simulink model "RELAY_TEST"  (Simulink 8.1)
settings: Solver=ode4  StartTime=0.0  StopTime=1.5  FixedStep=Ts  MaxStep=1e-3  RelTol=1e-3
model workspace (MAT data in the model file):
  op_snapshot1 : opcond.OperatingPoint (value not decoded)
PostLoadFcn:
  | Ts=100e-6; RELAY_TEST_init;
InitFcn:
  | Ts=100e-6; RELAY_TEST_init;
values from neighbouring files (symbols this model uses):
  cb_mech_delay = 5/60    (= 0.0833333333333)    [RELAY_TEST_init.m]
undefined symbols (not defined in the file or in its folder): cable_spec, Left, relay_par, type, V
libraries: rtlab x6, artemis x5, cables_lib x5, breaker_lib x3, relay_modbus_lib x3, rtio_generic_modbus x3, Load_lib x2, powerlib x2, ssn_lib x2, transformer_lib x2, powerlib_extras x1
settings Model: ARTEMISmethode_block_infos=$$__separator__$$RELAY_TEST/ARTEMIS Guide$$__separator__$$  Creator=RE25624  LastModifiedBy=re25624  BufferReuse=off
settings SolverCC: ZeroCrossAlgorithm=Adaptive
settings DataIOCC: ExternalInput=getinputstruct(op_snapshot1)  InitialState=getstatestruct(op_snapshot1)  LimitDataPoints=off  MaxDataPoints=90060  SignalLoggingSaveFormat=Dataset  SaveOutput=off  SignalLogging=off  DSMLogging=off  SaveTime=off  OutputSaveName=result
settings OptimizationCC: BlockReduction=off  OptimizeBlockIOStorage=off  BufferReuse=off  ExpressionFolding=off  LocalBlockOutputs=off
settings DebuggingCC: MaxConsecutiveZCsMsg=warning  IgnoredZcDiagnostic=none  SolverPrmCheckMsg=none  MultiTaskRateTransMsg=warning  FcnCallInpInsideContextMsg=EnableAllAsWarning  FrameProcessingCompatibilityMsg=error  ModelReferenceExtraNoncontSigs=warning  StrictBusMsg=None
settings ModelReferenceCC: UpdateModelReferenceTargets=IfOutOfDate
settings SFSimCC: SFSimEcho=off
settings GRTTargetCC: CodeReplacementLibrary=C89/C90 (ANSI)

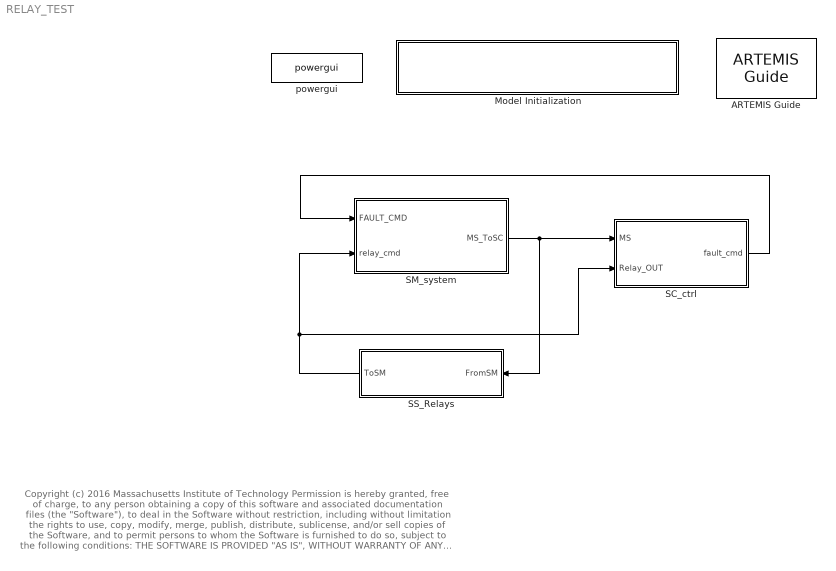
== system RELAY_TEST ==
  note: Copyright (c) 2016 Massachusetts Institute of Technology
      | Permission is hereby granted, free of charge, to any person obtaining a copy of this software and associated documentation files (the "Software"), to deal
      | in the Software without restriction, including without limitation the rights to use, copy, modify, merge, publish, distribute, sublicense, and/or sell copies of the
      | Software, and to permit persons to whom the Software is furnished to do so, subject to the following conditions:
      |
      | THE SOFTWARE IS PROVIDED "AS IS", WITHOUT WARRANTY OF ANY KIND, EXPRESS OR IMPLIED, INCLUDING BUT NOT LIMITED TO THE
      | WARRANTIES OF MERCHANTABILITY, FITNESS FOR A PARTICULAR PURPOSE AND NONINFRINGEMENT. IN NO EVENT SHALL THE AUTHORS
      | OR COPYRIGHT HOLDERS BE LIABLE FOR ANY CLAIM, DAMAGES OR OTHER LIABILITY, WHETHER IN AN ACTION OF CONTRACT, TORT OR
      | OTHERWISE, ARISING FROM, OUT OF OR IN CONNECTION WITH THE SOFTWARE OR THE USE OR OTHER DEALINGS IN THE SOFTWARE.
  ARTEMIS Guide : artemis/ARTEMIS/ARTEMIS Guide  Tag=FTSSmethode_opal_4hx0r99  Description=5.0_z1  lock=on  Ts=Ts  opt=art5  dyna=off  nb_perm=4  RT_fullcomp=off  ssn=on  ssn_itvc=off  ssn_ivic=off  ssn_ext=off  ssn_solver=Art5 with Backward Euler nodal interface  ssn_impulse=off  ssn_quasimpulse=off  ssn_impulse_loop=2  paraExtinctionThy=off  Thy_Impulse=on  dtc=Off  dtc_opt=normal  ao=on  simtype=off  ct_mac=off  lin_mov=off  lsp=[0.001 2]  spike_skip=Disabled  dtc_extra=1  dtc_sws=normal  dtc_pied=0.5  SPSRulesBlock=SPSRules  tre=on  ctmm=off  LF=off  dpl_type=ARTEMiS DPL  rlc_type=off  custom_type=off  para=on  ssn_ImpulseLoopBlockedStateUpdate=2  ssn_mov_iter_number=5  ssn_switch_iter_number=5
  Model Initialization : Subsystem  AncestorBlock=artemis/Tools /Misc/Model Initialization  mask(Model Functions){InitFcnX=Ts=100e-6; RELAY_TEST_init;, prel=off, posl=on, inif=on, strf=off}
      mask prompts: InitFcnX "Initialisation"; prel "Preload Function"; posl "PostLoad Function"; inif "InitFcn"; strf "StartFcn"
      mask init:
      | currentBlock = gcb;
      | root = bdroot(currentBlock);
      | 
      | 
      | if ~strcmp(get_param(root,'BlockDiagramType'),'library')
      |     if prel==1
      |         set_param(root, 'PreLoadFcn', InitFcnX);
      |     else
      |         set_param(root, 'PreLoadFcn', '');
      |     end
      |     if inif==1
      |         set_param(root, 'InitFcn', InitFcnX);
      |     else
      |         set_param(root, 'InitFcn', '');
      |     end
      |     if strf==1
      |         set_param(root, 'StartFcn', InitFcnX);
      |     else
      |         set_param(root, 'StartFcn', '');
      |     end
      |     if posl==1
      |         set_param(root, 'PostLoadFcn', InitFcnX);
      |     else
      |         set_param(root, 'PostLoadFcn', '');
      |     end
      | end
      | 
      | pos = get_param(currentBlock, 'Position');
      | width = pos(3) - pos(1); height = pos(4) - pos(2);
      | txt = [ upper(root) '\n' '- InitFcn. . . . . '  get_param(root, 'InitFcn') ];
      settings: CopyFcn=set_param(gcb,'LinkStatus','inactive')
      mask Display: text(5, height*0.5, txt, 'horizontalAlignment', 'left', 'verticalAlignment', 'middle') ;
  SC_ctrl : Subsystem
  SM_system : Subsystem
  SS_Relays : Subsystem
  powergui : powerlib/powergui  Priority=2  SimulationMode=Discrete  SolverType=Tustin  SampleTime=Ts  frequency=60  SPID=off  DisableSnubberDevices=off  DisableRonSwitches=off  DisableVfSwitches=off  SwTol=0  Interpol=off  DisplayEquations=off  frequencyindice=0  Pbase=100e6  ErrMax=1e-4  Iterations=50  UnitsV=kV  UnitsW=MW  FunctionMessages=off  echomessages=off  HookPort=off  EnableUseOfTLC=off  x0status=blocks  RestoreLinks=warning  ResistiveCurrentMeasurement=off  Frange=logspace(0,3,50)  Ylog=off  Xlog=off  ShowGrid=off  save=off  variable=ZData  structure=0  ZoomFFT=on  StartTime=0.0  cycles=2  DisplayStyle=off  fundamental=60  FreqAxis=off  MaxFrequency=1000  frequencyindicesteady=1  RmsSteady=1  display=off  Ts=0  methode=off
  wires:
  SM_system/1(MS_ToSC) -> SS_Relays/1(FromSM), SC_ctrl/1(MS)
  SS_Relays/1(ToSM) -> SM_system/2(relay_cmd), SC_ctrl/2(Relay_OUT)
  SC_ctrl/1(fault_cmd) -> SM_system/1(FAULT_CMD)

== system RELAY_TEST/Model Initialization ==

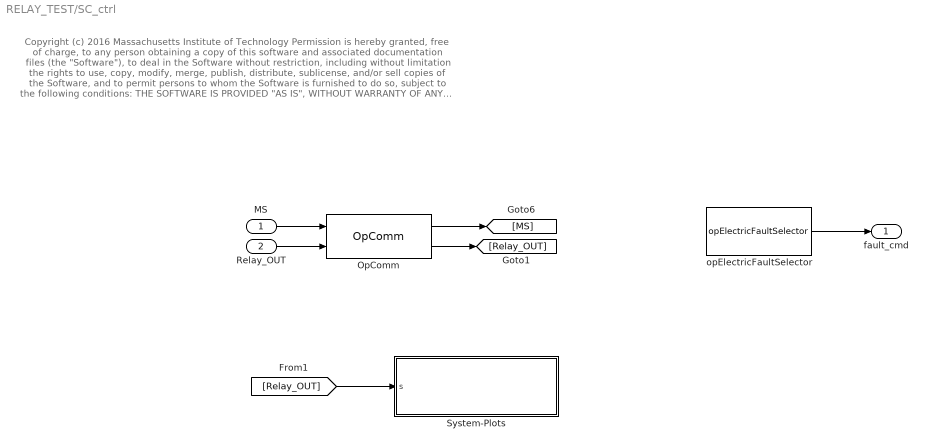
== system RELAY_TEST/SC_ctrl ==
  note: Copyright (c) 2016 Massachusetts Institute of Technology
      | Permission is hereby granted, free of charge, to any person obtaining a copy of this software and associated documentation files (the "Software"), to deal
      | in the Software without restriction, including without limitation the rights to use, copy, modify, merge, publish, distribute, sublicense, and/or sell copies of the
      | Software, and to permit persons to whom the Software is furnished to do so, subject to the following conditions:
      |
      | THE SOFTWARE IS PROVIDED "AS IS", WITHOUT WARRANTY OF ANY KIND, EXPRESS OR IMPLIED, INCLUDING BUT NOT LIMITED TO THE
      | WARRANTIES OF MERCHANTABILITY, FITNESS FOR A PARTICULAR PURPOSE AND NONINFRINGEMENT. IN NO EVENT SHALL THE AUTHORS
      | OR COPYRIGHT HOLDERS BE LIABLE FOR ANY CLAIM, DAMAGES OR OTHER LIABILITY, WHETHER IN AN ACTION OF CONTRACT, TORT OR
      | OTHERWISE, ARISING FROM, OUT OF OR IN CONNECTION WITH THE SOFTWARE OR THE USE OR OTHER DEALINGS IN THE SOFTWARE.
  MS : Inport
  Relay_OUT : Inport  Port=2
  OpComm : rtlab/OpComm  nbport=2  groupe_acq=1  subsys_rate=0  st=0  Synchronization=on  Interpolation=on  Threshold=1.0  Missed_Data=off  Sim_Time=off  Samples=off  dynSigOut=off  from_console=0  warning_done=off  writeOpCommFile=off  Offset=off
  System-Plots : Subsystem
  opElectricFaultSelector : artemis/Tools /POW faults/opElectricFaultSelector  phase_a=on  phase_b=on  phase_c=on  gnd_fault=on  Tacq=1  Tst=[0.1 0 10]  enable_POW=on  angle_POW=[15 0 10]  Tdr="[10.5 0  20]"  fault_location_menu=location 2  T_init=0
  fault_cmd : Outport
  wires:
  OpComm/1 -> [MS]
  MS/1 -> OpComm/1
  OpComm/2 -> [Relay_OUT]
  Relay_OUT/1 -> OpComm/2
  opElectricFaultSelector/1 -> fault_cmd/1
  [Relay_OUT] -> System-Plots/1(s)

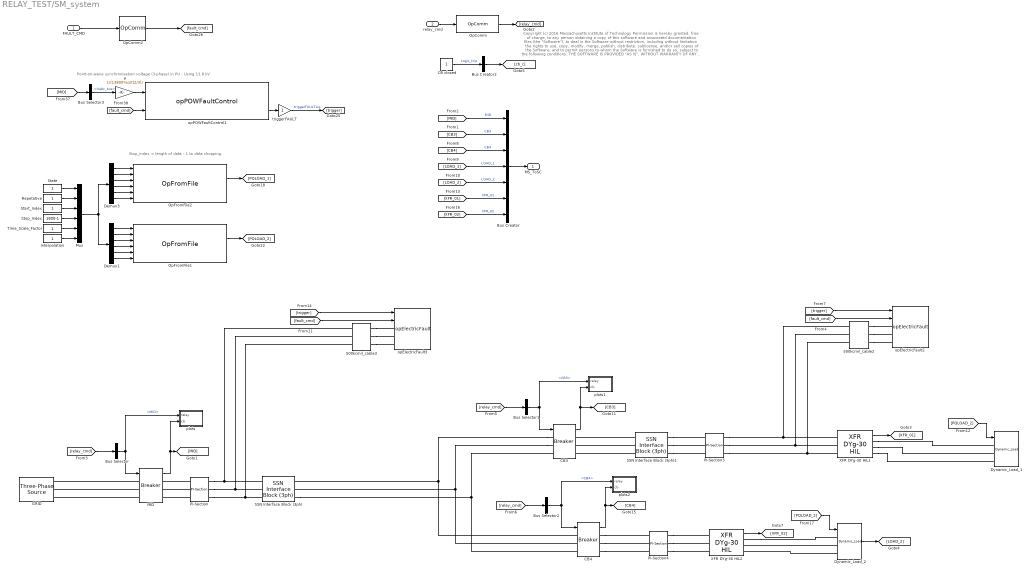
== system RELAY_TEST/SM_system ==
  note: Copyright (c) 2016 Massachusetts Institute of Technology
      | Permission is hereby granted, free of charge, to any person obtaining a copy of this software and associated documentation files (the "Software"), to deal
      | in the Software without restriction, including without limitation the rights to use, copy, modify, merge, publish, distribute, sublicense, and/or sell copies of the
      | Software, and to permit persons to whom the Software is furnished to do so, subject to the following conditions:
      |
      | THE SOFTWARE IS PROVIDED "AS IS", WITHOUT WARRANTY OF ANY KIND, EXPRESS OR IMPLIED, INCLUDING BUT NOT LIMITED TO THE
      | WARRANTIES OF MERCHANTABILITY, FITNESS FOR A PARTICULAR PURPOSE AND NONINFRINGEMENT. IN NO EVENT SHALL THE AUTHORS
      | OR COPYRIGHT HOLDERS BE LIABLE FOR ANY CLAIM, DAMAGES OR OTHER LIABILITY, WHETHER IN AN ACTION OF CONTRACT, TORT OR
      | OTHERWISE, ARISING FROM, OUT OF OR IN CONNECTION WITH THE SOFTWARE OR THE USE OR OTHER DEALINGS IN THE SOFTWARE
  note: Stop_index = length of data - 1 to data chopping
  note: Point-on-wave synchronisation voltage (3-phase) in PU - Using 13.8 kV
  FAULT_CMD : Inport
  relay_cmd : Inport  Port=2
  500kcmil_cable2 : cables_lib/500kcmil_cable  length=1  par_sets=1
  500kcmil_cable3 : cables_lib/500kcmil_cable  length=1  par_sets=1
  Bus Creator : BusCreator  Inputs=7
  Bus Creator2 : BusCreator  Inputs=1
  Bus Selector : BusSelector  OutputSignals=MID
  Bus Selector1 : BusSelector  OutputSignals=CB3
  Bus Selector2 : BusSelector  OutputSignals=CB4
  Bus Selector3 : BusSelector  OutputSignals=Vabc_bus
  CB closed : Constant
  CB3 : breaker_lib/Breaker  Ts=Ts  mech_delays=[cb_mech_delay(1,:)]
  CB4 : breaker_lib/Breaker  Ts=Ts  mech_delays=[cb_mech_delay(1,:)]
  Demux1 : Demux  Outputs=6
  Demux3 : Demux  Outputs=6
  Dynamic_Load_1 : Load_lib/Dynamic_Load  V=4160  Ts=Ts
  Dynamic_Load_2 : Load_lib/Dynamic_Load  V=480  Ts=Ts
  GRID : powerlib/Electrical Sources/Three-Phase Source  Voltage=13800  PhaseAngle=0  Frequency=60  InternalConnection=Yg  SpecifyImpedance=on  Resistance=0.8929  Inductance=16.58e-3  ShortCircuitLevel=375e6  BaseVoltage=13800  XRratio=4.6  BusType=swing  Pref=0  Qref=0  Qmin=-inf  Qmax=inf
  "Interpolation " : Constant
  MID : breaker_lib/Breaker  Ts=Ts  mech_delays=[cb_mech_delay(1,:)]
  Mux : Mux  Inputs=6
  OpComm : rtlab/OpComm  nbport=1  groupe_acq=1  subsys_rate=0  st=0  Synchronization=on  Interpolation=on  Threshold=1.0  Missed_Data=off  Sim_Time=off  Samples=off  dynSigOut=off  from_console=0  warning_done=off  writeOpCommFile=off  Offset=off
  OpComm2 : rtlab/OpComm  nbport=1  groupe_acq=1  subsys_rate=0  st=0  Synchronization=on  Interpolation=on  Threshold=1.0  Missed_Data=off  Sim_Time=off  Samples=off  dynSigOut=off  from_console=1  warning_done=off  writeOpCommFile=off  Offset=off
  OpFromFile1 : rtlab/DataLogging/OpFromFile  filename_mode=Static (same filename all the time)  reload_mode=Next time model is paused (Real-Time)  init_file_id=0  filename=one_min_data.mat  rtpath='./'  nrtpath='.\'  sample_time=0
  OpFromFile2 : rtlab/DataLogging/OpFromFile  filename_mode=Static (same filename all the time)  reload_mode=Next time model is paused (Real-Time)  init_file_id=0  filename=one_min_data.mat  rtpath='./'  nrtpath='.\'  sample_time=0
  PI-Section : cables_lib/PI-Section  cable_spec=[cable_spec(13, :)]  line_length=5500  parallel_sets=1
  PI-Section3 : cables_lib/PI-Section  cable_spec=[cable_spec(13, :)]  line_length=1500  parallel_sets=1
  PI-Section4 : cables_lib/PI-Section  cable_spec=[cable_spec(13, :)]  line_length=7000  parallel_sets=1
  "Repetative " : Constant
  SSN Interface Block (3ph) : ssn_lib/SSN Interface Block (3ph)  nb_phase=3  nb_port=2  p1_type=V-type(Left)  p2_type=V-type (Right)  p3_type=V-type(Left)  p4_type=V-type(Left)  p5_type=V-type(Left)  p6_type=V-type(Left)  p7_type=V-type(Left)  p8_type=V-type(Left)  p9_type=V-type(Left)  p10_type=V-type(Left)  p11_type=V-type(Left)  p12_type=V-type(Left)  p13_type=V-type(Left)  p14_type=V-type(Left)  p15_type=V-type(Left)  p16_type=V-type(Left)  I_port_shunt_resistance=1e9
  SSN Interface Block (3ph)1 : ssn_lib/SSN Interface Block (3ph)  nb_phase=3  nb_port=2  p1_type=V-type(Left)  p2_type=V-type (Right)  p3_type=V-type(Left)  p4_type=V-type(Left)  p5_type=V-type(Left)  p6_type=V-type(Left)  p7_type=V-type(Left)  p8_type=V-type(Left)  p9_type=V-type(Left)  p10_type=V-type(Left)  p11_type=V-type(Left)  p12_type=V-type(Left)  p13_type=V-type(Left)  p14_type=V-type(Left)  p15_type=V-type(Left)  p16_type=V-type(Left)  I_port_shunt_resistance=1e9
  "Start_Index " : Constant
  "State " : Constant
  "Stop_Index " : Constant  Value=1800-1
  "Time_Scale_Factor " : Constant
  XFR DYg-30 HIL1 : transformer_lib/XFR DYg-30 HIL  Rating=3750  Vp=13800  Vs=4160  Z=4.75  XR=11.4
  XFR DYg-30 HIL2 : transformer_lib/XFR DYg-30 HIL  Rating=2500  Vp=13800  Vs=480  Z=5.75  XR=6.6
  a : Gain  Gain=1/(13800*sqrt(2/3))
  opElectricFault2 : artemis/Tools /POW faults/opElectricFault  FaultLocation=location 2  FaultResistance=0.0001  GroundResistance=0.0001  InitialStates=[0 0 0]  SnubberResistance=1e6  SnubberCapacitance=inf
  opElectricFault3 : artemis/Tools /POW faults/opElectricFault  FaultLocation=location 1  FaultResistance=0.0001  GroundResistance=0.0001  InitialStates=[0 0 0]  SnubberResistance=1e6  SnubberCapacitance=inf
  opPOWFaultControl1 : artemis/Tools /POW faults/opPOWFaultControl  Ts=Ts  usePLL=off  Fgrid=60  PLL_k=[180 3200 1]  vol_sel=1: rising zero-corssing  SyncPhase_menu=A  T_acq=0.8
  plots : Subsystem
  plots1 : Subsystem
  plots2 : Subsystem
  triggerFAULT : Gain
  MS_ToSC : Outport
  wires:
  MID/1 -> plots/2(cb), [MID]
  Bus Creator/1 -> MS_ToSC/1
  OpComm/1 -> [relay_cmd]
  relay_cmd/1 -> OpComm/1
  XFR DYg-30 HIL1/1 -> [XFR_01]
  "Stop_Index "/1 -> Mux/4
  Demux1/2 -> OpFromFile1/2
  Demux1/5 -> OpFromFile1/5
  OpFromFile1/2 -> [PQLOAD_2]
  "Interpolation "/1 -> Mux/6
  Demux1/4 -> OpFromFile1/4
  Demux1/1 -> OpFromFile1/1
  Demux1/6 -> OpFromFile1/6
  Demux1/3 -> OpFromFile1/3
  "Start_Index "/1 -> Mux/3
  "Time_Scale_Factor "/1 -> Mux/5
  "Repetative "/1 -> Mux/2
  "State "/1 -> Mux/1
  XFR DYg-30 HIL2/1 -> [XFR_02]
  Bus Creator2/1 -> [cb_c]
  CB closed/1 -> Bus Creator2/1  "Logic_trip"
  [XFR_02] -> Bus Creator/7  "XFR_02"
  [LOAD_2] -> Bus Creator/5  "LOAD_2"
  [XFR_01] -> Bus Creator/6  "XFR_01"
  [MID] -> Bus Creator/1  "MID"
  [CB4] -> Bus Creator/3  "CB4"
  [CB3] -> Bus Creator/2  "CB3"
  [LOAD_1] -> Bus Creator/4  "LOAD_1"
  Demux3/2 -> OpFromFile2/2
  Demux3/5 -> OpFromFile2/5
  OpFromFile2/2 -> [PQLOAD_1]
  Demux3/4 -> OpFromFile2/4
  Demux3/1 -> OpFromFile2/1
  Demux3/6 -> OpFromFile2/6
  Demux3/3 -> OpFromFile2/3
  Mux/1 -> Demux1/1, Demux3/1
  [relay_cmd] -> Bus Selector/1
  Bus Selector/1 -> plots/1(relay), MID/1  "<MID>"
  [relay_cmd] -> Bus Selector1/1
  [relay_cmd] -> Bus Selector2/1
  [fault_cmd] -> opPOWFaultControl1/2
  opPOWFaultControl1/2 -> triggerFAULT/1
  triggerFAULT/1 -> [trigger]  "triggerFAULTsig"
  [MID] -> Bus Selector3/1
  Bus Selector3/1 -> a/1  "<Vabc_bus>"
  a/1 -> opPOWFaultControl1/1
  OpComm2/1 -> [fault_cmd]
  FAULT_CMD/1 -> OpComm2/1
  [fault_cmd] -> opElectricFault2/2
  [trigger] -> opElectricFault2/1
  [fault_cmd] -> opElectricFault3/2
  [trigger] -> opElectricFault3/1
  CB3/1 -> [CB3], plots1/2(cb)
  Bus Selector1/1 -> CB3/1, plots1/1(relay)  "<CB3>"
  CB4/1 -> plots2/2(cb), [CB4]
  Bus Selector2/1 -> CB4/1, plots2/1(relay)  "<CB4>"
  Dynamic_Load_2/1 -> [LOAD_2]
  [PQLOAD_2] -> Dynamic_Load_2/1
  [PQLOAD_2] -> Dynamic_Load_1/1
  connections:
  CB4/RConn2 -- PI-Section4/LConn2
  CB4/RConn1 -- PI-Section4/LConn1
  CB4/RConn3 -- PI-Section4/LConn3
  PI-Section4/RConn1 -- XFR DYg-30 HIL2/LConn1
  PI-Section4/RConn2 -- XFR DYg-30 HIL2/LConn2
  PI-Section4/RConn3 -- XFR DYg-30 HIL2/LConn3
  PI-Section3/RConn2 -- 500kcmil_cable2/LConn2 -- XFR DYg-30 HIL1/LConn2
  PI-Section3/RConn3 -- 500kcmil_cable2/LConn3 -- XFR DYg-30 HIL1/LConn3
  PI-Section3/RConn1 -- 500kcmil_cable2/LConn1 -- XFR DYg-30 HIL1/LConn1
  500kcmil_cable2/RConn2 -- opElectricFault2/LConn2
  500kcmil_cable2/RConn1 -- opElectricFault2/LConn1
  500kcmil_cable2/RConn3 -- opElectricFault2/LConn3
  500kcmil_cable3/RConn2 -- opElectricFault3/LConn2
  500kcmil_cable3/RConn1 -- opElectricFault3/LConn1
  500kcmil_cable3/RConn3 -- opElectricFault3/LConn3
  SSN Interface Block (3ph)1/RConn2 -- PI-Section3/LConn2
  SSN Interface Block (3ph)1/RConn1 -- PI-Section3/LConn1
  SSN Interface Block (3ph)1/RConn3 -- PI-Section3/LConn3
  SSN Interface Block (3ph)1/LConn3 -- CB3/RConn3
  SSN Interface Block (3ph)1/LConn1 -- CB3/RConn1
  SSN Interface Block (3ph)1/LConn2 -- CB3/RConn2
  500kcmil_cable3/LConn1 -- SSN Interface Block (3ph)/LConn1 -- PI-Section/RConn1
  500kcmil_cable3/LConn2 -- SSN Interface Block (3ph)/LConn2 -- PI-Section/RConn2
  500kcmil_cable3/LConn3 -- SSN Interface Block (3ph)/LConn3 -- PI-Section/RConn3
  SSN Interface Block (3ph)/RConn3 -- CB3/LConn3 -- CB4/LConn3
  CB3/LConn1 -- SSN Interface Block (3ph)/RConn1 -- CB4/LConn1
  CB3/LConn2 -- SSN Interface Block (3ph)/RConn2 -- CB4/LConn2
  Dynamic_Load_2/LConn2 -- XFR DYg-30 HIL2/RConn2
  Dynamic_Load_2/LConn3 -- XFR DYg-30 HIL2/RConn3
  Dynamic_Load_2/LConn1 -- XFR DYg-30 HIL2/RConn1
  XFR DYg-30 HIL1/RConn1 -- Dynamic_Load_1/LConn1
  XFR DYg-30 HIL1/RConn2 -- Dynamic_Load_1/LConn2
  XFR DYg-30 HIL1/RConn3 -- Dynamic_Load_1/LConn3
  PI-Section/LConn2 -- MID/RConn2
  PI-Section/LConn1 -- MID/RConn1
  PI-Section/LConn3 -- MID/RConn3
  MID/LConn1 -- GRID/RConn1
  MID/LConn2 -- GRID/RConn2
  MID/LConn3 -- GRID/RConn3

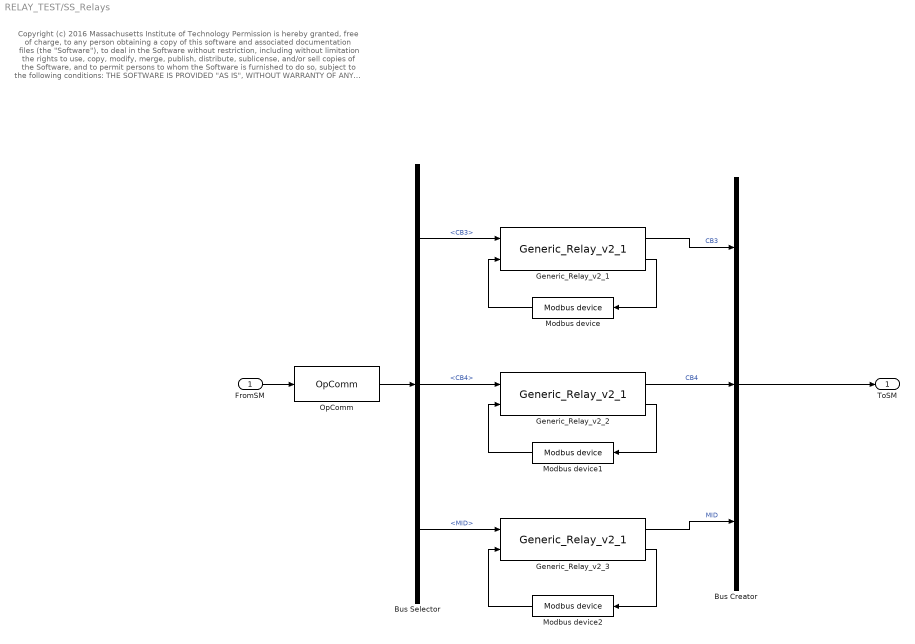
== system RELAY_TEST/SS_Relays ==
  note: Copyright (c) 2016 Massachusetts Institute of Technology
      | Permission is hereby granted, free of charge, to any person obtaining a copy of this software and associated documentation files (the "Software"), to deal
      | in the Software without restriction, including without limitation the rights to use, copy, modify, merge, publish, distribute, sublicense, and/or sell copies of the
      | Software, and to permit persons to whom the Software is furnished to do so, subject to the following conditions:
      |
      | THE SOFTWARE IS PROVIDED "AS IS", WITHOUT WARRANTY OF ANY KIND, EXPRESS OR IMPLIED, INCLUDING BUT NOT LIMITED TO THE
      | WARRANTIES OF MERCHANTABILITY, FITNESS FOR A PARTICULAR PURPOSE AND NONINFRINGEMENT. IN NO EVENT SHALL THE AUTHORS
      | OR COPYRIGHT HOLDERS BE LIABLE FOR ANY CLAIM, DAMAGES OR OTHER LIABILITY, WHETHER IN AN ACTION OF CONTRACT, TORT OR
      | OTHERWISE, ARISING FROM, OUT OF OR IN CONNECTION WITH THE SOFTWARE OR THE USE OR OTHER DEALINGS IN THE SOFTWARE
  FromSM : Inport
  Bus Creator : BusCreator  Inputs=3
  Bus Selector : BusSelector  OutputSignals=CB3,CB4,MID
  Generic_Relay_v2_1 : relay_modbus_lib/Generic_Relay_v2_1  Ts=Ts  relay_settings=[relay_par(1,:)]
  Generic_Relay_v2_2 : relay_modbus_lib/Generic_Relay_v2_1  Ts=Ts  relay_settings=[relay_par(2,:)]
  Generic_Relay_v2_3 : relay_modbus_lib/Generic_Relay_v2_1  Ts=Ts  relay_settings=[relay_par(1,:)]
  Modbus device : rtio_generic_modbus/Modbus device  conf_name=F1_relay_cfg1.opal  conf_name_mask=F1_relay_cfg1.xls  sample_time=Ts
  Modbus device1 : rtio_generic_modbus/Modbus device  conf_name=F1_relay_cfg2.opal  conf_name_mask=F1_relay_cfg2.xls  sample_time=Ts
  Modbus device2 : rtio_generic_modbus/Modbus device  conf_name=F1_relay_cfg3.opal  conf_name_mask=F1_relay_cfg3.xls  sample_time=Ts
  OpComm : rtlab/OpComm  nbport=1  groupe_acq=1  subsys_rate=0  st=0  Synchronization=on  Interpolation=on  Threshold=1.0  Missed_Data=off  Sim_Time=off  Samples=off  dynSigOut=off  from_console=0  warning_done=off  writeOpCommFile=off  Offset=off
  ToSM : Outport
  wires:
  OpComm/1 -> Bus Selector/1
  FromSM/1 -> OpComm/1
  Generic_Relay_v2_1/1 -> Bus Creator/1  "CB3"
  Generic_Relay_v2_2/1 -> Bus Creator/2  "CB4"
  Bus Creator/1 -> ToSM/1
  Generic_Relay_v2_3/1 -> Bus Creator/3  "MID"
  Bus Selector/1 -> Generic_Relay_v2_1/1  "<CB3>"
  Bus Selector/2 -> Generic_Relay_v2_2/1  "<CB4>"
  Bus Selector/3 -> Generic_Relay_v2_3/1  "<MID>"
  Modbus device/1 -> Generic_Relay_v2_1/2
  Generic_Relay_v2_1/2 -> Modbus device/1
  Modbus device1/1 -> Generic_Relay_v2_2/2
  Generic_Relay_v2_2/2 -> Modbus device1/1
  Modbus device2/1 -> Generic_Relay_v2_3/2
  Generic_Relay_v2_3/2 -> Modbus device2/1

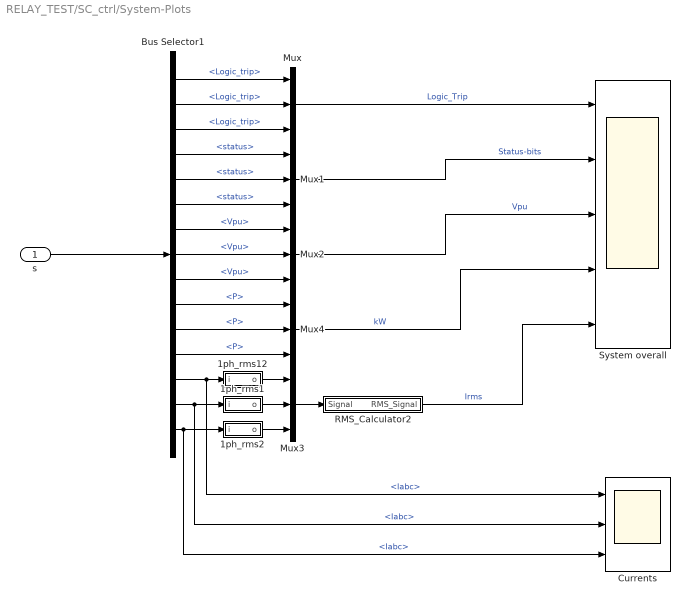
== system RELAY_TEST/SC_ctrl/System-Plots ==
  s : Inport
  1ph_rms1 : Subsystem
  1ph_rms12 : Subsystem
  1ph_rms2 : Subsystem
  Bus Selector1 : BusSelector  OutputSignals=CB3.Logic_trip,CB4.Logic_trip,MID.Logic_trip,CB3.m.status,CB4.m.status,MID.m.status,CB3.m.Vpu,CB4.m.Vpu,MID.m.Vpu,CB3.m.P,CB4.m.P,MID.m.P,CB3.m.Iabc,CB4.m.Iabc,MID.m.Iabc
  Currents : Scope  NumInputPorts=3
      settings: ShowLegends=on  TimeRange=0.5  YMin=-1~-1~-200  YMax=1~1~200
  Mux{,1..4} (5 alike) : Mux  Inputs=3
  RMS_Calculator2 : Subsystem
  System overall : Scope  NumInputPorts=5
      settings: ShowLegends=on  TimeRange=4.5  YMin=0~0~0~-10000000~0  YMax=1~20~1.4~50000000~10000
  wires:
  s/1 -> Bus Selector1/1
  Bus Selector1/11 -> Mux4/2  "<P>"
  Bus Selector1/3 -> Mux/3  "<Logic_trip>"
  Bus Selector1/5 -> Mux1/2  "<status>"
  Bus Selector1/9 -> Mux2/3  "<Vpu>"
  Bus Selector1/14 -> Currents/2, 1ph_rms1/1(i)  "<Iabc>"
  Bus Selector1/2 -> Mux/2  "<Logic_trip>"
  Bus Selector1/6 -> Mux1/3  "<status>"
  Bus Selector1/12 -> Mux4/3  "<P>"
  Bus Selector1/1 -> Mux/1  "<Logic_trip>"
  Bus Selector1/10 -> Mux4/1  "<P>"
  Bus Selector1/7 -> Mux2/1  "<Vpu>"
  Bus Selector1/4 -> Mux1/1  "<status>"
  Bus Selector1/8 -> Mux2/2  "<Vpu>"
  Bus Selector1/13 -> Currents/1, 1ph_rms12/1(i)  "<Iabc>"
  Bus Selector1/15 -> Currents/3, 1ph_rms2/1(i)  "<Iabc>"
  1ph_rms2/1(o) -> Mux3/3
  Mux2/1 -> System overall/3  "Vpu"
  Mux1/1 -> System overall/2  "Status-bits"
  Mux4/1 -> System overall/4  "kW"
  RMS_Calculator2/1(RMS_Signal) -> System overall/5  "Irms"
  Mux/1 -> System overall/1  "Logic_Trip"
  Mux3/1 -> RMS_Calculator2/1(Signal)
  1ph_rms1/1(o) -> Mux3/2
  1ph_rms12/1(o) -> Mux3/1

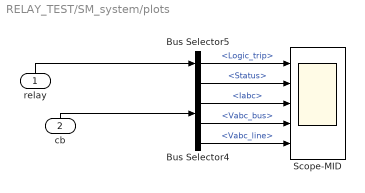
== system RELAY_TEST/SM_system/plots ==
  relay : Inport
  cb : Inport  Port=2
  Bus Selector4 : BusSelector  OutputSignals=Status,Iabc,Vabc_bus,Vabc_line
  Bus Selector5 : BusSelector  OutputSignals=Logic_trip
  Scope-MID : Scope  NumInputPorts=5
      settings: TimeRange=1.5  YMin=0~0~-20000~-30000~-15000  YMax=1~1~15000~30000~15000  SaveName=ScopeData3
  wires:
  cb/1 -> Bus Selector4/1
  relay/1 -> Bus Selector5/1
  Bus Selector4/2 -> Scope-MID/3  "<Iabc>"
  Bus Selector4/3 -> Scope-MID/4  "<Vabc_bus>"
  Bus Selector4/1 -> Scope-MID/2  "<Status>"
  Bus Selector4/4 -> Scope-MID/5  "<Vabc_line>"
  Bus Selector5/1 -> Scope-MID/1  "<Logic_trip>"

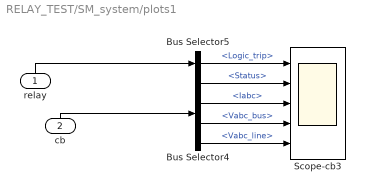
== system RELAY_TEST/SM_system/plots1 ==
  relay : Inport
  cb : Inport  Port=2
  Bus Selector4 : BusSelector  OutputSignals=Status,Iabc,Vabc_bus,Vabc_line
  Bus Selector5 : BusSelector  OutputSignals=Logic_trip
  Scope-cb3 : Scope  NumInputPorts=5
      settings: TimeRange=1.5  YMin=0~0~-20000~-15000~-15000  YMax=1~1~15000~15000~15000  SaveName=ScopeData3
  wires:
  cb/1 -> Bus Selector4/1
  relay/1 -> Bus Selector5/1
  Bus Selector4/2 -> Scope-cb3/3  "<Iabc>"
  Bus Selector4/3 -> Scope-cb3/4  "<Vabc_bus>"
  Bus Selector4/1 -> Scope-cb3/2  "<Status>"
  Bus Selector4/4 -> Scope-cb3/5  "<Vabc_line>"
  Bus Selector5/1 -> Scope-cb3/1  "<Logic_trip>"

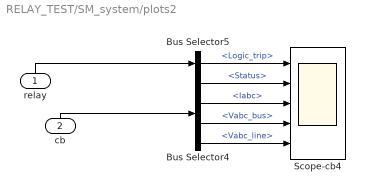
== system RELAY_TEST/SM_system/plots2 ==
  relay : Inport
  cb : Inport  Port=2
  Bus Selector4 : BusSelector  OutputSignals=Status,Iabc,Vabc_bus,Vabc_line
  Bus Selector5 : BusSelector  OutputSignals=Logic_trip
  Scope-cb4 : Scope  NumInputPorts=5
      settings: TimeRange=1.5  YMin=0~0~-200~-15000~-15000  YMax=1~1~200~15000~15000  SaveName=ScopeData3
  wires:
  cb/1 -> Bus Selector4/1
  relay/1 -> Bus Selector5/1
  Bus Selector4/2 -> Scope-cb4/3  "<Iabc>"
  Bus Selector4/3 -> Scope-cb4/4  "<Vabc_bus>"
  Bus Selector4/1 -> Scope-cb4/2  "<Status>"
  Bus Selector4/4 -> Scope-cb4/5  "<Vabc_line>"
  Bus Selector5/1 -> Scope-cb4/1  "<Logic_trip>"

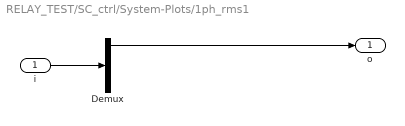
== system RELAY_TEST/SC_ctrl/System-Plots/1ph_rms1 ==
  i : Inport
  Demux : Demux  Outputs=3
  o : Outport
  wires:
  i/1 -> Demux/1
  Demux/1 -> o/1

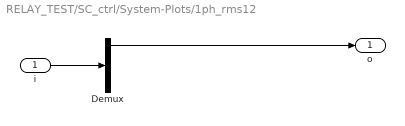
== system RELAY_TEST/SC_ctrl/System-Plots/1ph_rms12 ==
  i : Inport
  Demux : Demux  Outputs=3
  o : Outport
  wires:
  i/1 -> Demux/1
  Demux/1 -> o/1

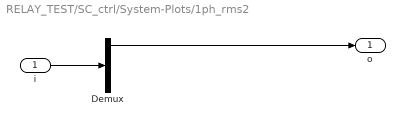
== system RELAY_TEST/SC_ctrl/System-Plots/1ph_rms2 ==
  i : Inport
  Demux : Demux  Outputs=3
  o : Outport
  wires:
  i/1 -> Demux/1
  Demux/1 -> o/1

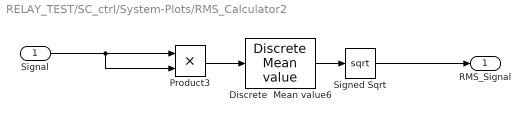
== system RELAY_TEST/SC_ctrl/System-Plots/RMS_Calculator2 ==
  Signal : Inport
  Discrete  Mean value6 : powerlib_extras/Discrete Measurements/Discrete  Mean value  Freq=60  Vinit=0  Ts=Ts
  Product3 : Product  RndMeth=Zero
  Signed Sqrt : Sqrt  SaturateOnIntegerOverflow=on
  RMS_Signal : Outport
  wires:
  Signal/1 -> Product3/1, Product3/2
  Product3/1 -> Discrete  Mean value6/1
  Discrete  Mean value6/1 -> Signed Sqrt/1
  Signed Sqrt/1 -> RMS_Signal/1
